simulink library "time_conversion_lib"  (R2016b)
settings: Solver=ode45  StartTime=0.0  StopTime=10.0  RelTol=1e-3  EnableMultiTasking=on
settings Model: Creator=Taylor  LastModifiedBy=taylorreynolds
settings DataIOCC: LimitDataPoints=on
settings OptimizationCC: LifeSpan=inf
settings DebuggingCC: AllowSymbolicDim=off  SFUnexpectedBacktrackingDiag=warning  SFNoUnconditionalDefaultTransitionDiag=warning  SFExecutionAtInitializationDiag=none
settings GRTTargetCC: TargetLangStandard=C89/C90 (ANSI)  GeneratePreprocessorConditionals=Disable all
settings ConfigComp: CovMetricSettings=dw  CovHtmlReporting=on  CovSaveCumulativeToWorkspaceVar=on  CovSaveSingleToWorkspaceVar=on  CovExternalEMLEnable=off

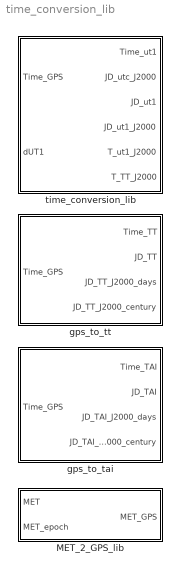
== system time_conversion_lib ==
  MET_2_GPS_lib : Subsystem
  gps_to_tai : Subsystem
  gps_to_tt : Subsystem
  time_conversion_lib : Subsystem

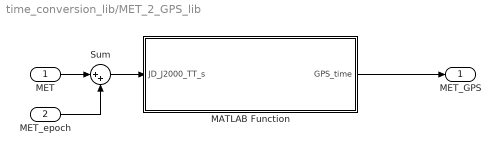
== system time_conversion_lib/MET_2_GPS_lib ==
  MET : Inport
  MET_epoch : Inport  Port=2
  MATLAB Function : MATLAB Function  TreatAsAtomicUnit=on
  Sum : Sum  Inputs=|++
  MET_GPS : Outport
  wires:
  MATLAB Function/1(GPS_time) -> MET_GPS/1
  MET/1 -> Sum/1
  MET_epoch/1 -> Sum/2
  Sum/1 -> MATLAB Function/1(JD_J2000_TT_s)

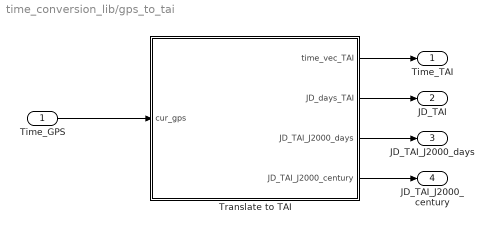
== system time_conversion_lib/gps_to_tai ==
  Time_GPS : Inport
  Translate to TAI : MATLAB Function  TreatAsAtomicUnit=on
  Time_TAI : Outport
  JD_TAI : Outport  Port=2
  JD_TAI_J2000_days : Outport  Port=3
  JD_TAI_J2000_century : Outport  Port=4
  wires:
  Translate to TAI/3(JD_TAI_J2000_days) -> JD_TAI_J2000_days/1
  Time_GPS/1 -> Translate to TAI/1(cur_gps)
  Translate to TAI/1(time_vec_TAI) -> Time_TAI/1
  Translate to TAI/2(JD_days_TAI) -> JD_TAI/1
  Translate to TAI/4(JD_TAI_J2000_century) -> JD_TAI_J2000_century/1

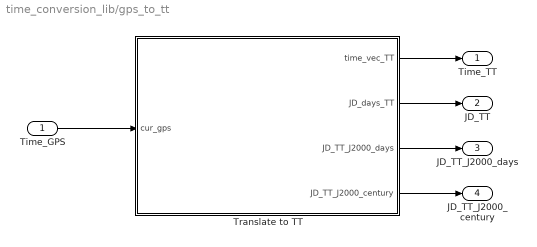
== system time_conversion_lib/gps_to_tt ==
  Time_GPS : Inport
  Translate to TT : MATLAB Function  TreatAsAtomicUnit=on
  Time_TT : Outport
  JD_TT : Outport  Port=2
  JD_TT_J2000_days : Outport  Port=3
  JD_TT_J2000_century : Outport  Port=4
  wires:
  Time_GPS/1 -> Translate to TT/1(cur_gps)
  Translate to TT/1(time_vec_TT) -> Time_TT/1
  Translate to TT/2(JD_days_TT) -> JD_TT/1
  Translate to TT/3(JD_TT_J2000_days) -> JD_TT_J2000_days/1
  Translate to TT/4(JD_TT_J2000_century) -> JD_TT_J2000_century/1

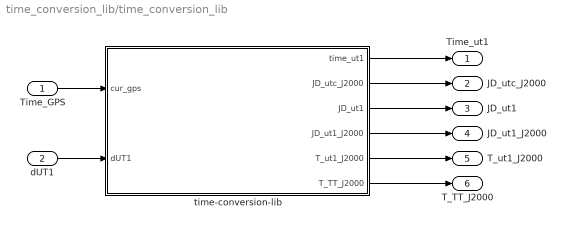
== system time_conversion_lib/time_conversion_lib ==
  Time_GPS : Inport
  dUT1 : Inport  Port=2
  time-conversion-lib : MATLAB Function  TreatAsAtomicUnit=on
  Time_ut1 : Outport
  JD_utc_J2000 : Outport  Port=2
  JD_ut1 : Outport  Port=3
  JD_ut1_J2000 : Outport  Port=4
  T_ut1_J2000 : Outport  Port=5
  T_TT_J2000 : Outport  Port=6
  wires:
  dUT1/1 -> time-conversion-lib/2(dUT1)
  time-conversion-lib/4(JD_ut1_J2000) -> JD_ut1_J2000/1
  Time_GPS/1 -> time-conversion-lib/1(cur_gps)
  time-conversion-lib/1(time_ut1) -> Time_ut1/1
  time-conversion-lib/5(T_ut1_J2000) -> T_ut1_J2000/1
  time-conversion-lib/3(JD_ut1) -> JD_ut1/1
  time-conversion-lib/6(T_TT_J2000) -> T_TT_J2000/1
  time-conversion-lib/2(JD_utc_J2000) -> JD_utc_J2000/1

== matlab function time_conversion_lib/gps_to_tai/Translate to TAI ==
  data: cur_gps input; time_vec_TAI output; JD_days_TAI output; JD_TAI_J2000_days output; JD_TAI_J2000_century output
function [time_vec_TAI,JD_days_TAI,JD_TAI_J2000_days,JD_TAI_J2000_century] = fcn(cur_gps)
% ----------------------------------------------------------------------- %
% Husky-Sat 1, ADCS Subsystem
% T. Reynolds -- 2.7.18
% 
% Convert a GPS time into date-time, Julian date and Julian century in the
% TAI frame. Accounts for leap seconds, and uses both the regular JD epoch
% and J2000.
%
% #codegen
% ------ Constants ------ %
% Account for dUT1 to get closest estimate to UT1
%   dUT1 obtained from:
%       http://maia.usno.navy.mil/ser7/finals.daily
% ----------------------------------------------------------------------- %

% Constants
gps2tai     = 19; % Account for leap seconds GPS --> TAI
sec2day     = 1/86400; 
day2sec     = 86400;
week2day    = 7;
JD_1900     = 2415019.5;
JD_GPSepoch = 2444244.5;
JD_J2000    = 2451545.0;
JD2cent     = 1/36525;
Lmonth      = [31, 28, 31, 30, 31, 30, 31, 31, 30, 31, 30, 31];

sec_in = cur_gps(1); week_in = cur_gps(2);
% --------------------------- %

% Translate GPS w-s to JD and Gregorian ymd-hms
JD_days_gps     = JD_GPSepoch + week2day*week_in + sec2day*sec_in;
JD_days_TAI     = JD_days_gps + sec2JD*gps2tai;

JD_TAI_J2000_days       = JD_days_TAI - JD_J2000;
JD_TAI_J2000_century    = JD_TAI_J2000_days*JD2cent;

T1900   = (JD_days_TAI - JD_1900)/365.25;

year    = 1900 + floor(T1900);

leapyrs     = floor((year - 1900 - 1)*0.25);
days    = (JD_days_TAI - JD_1900) - ((year - 1900)*365 + leapyrs );

if days < 1
    year = year - 1;
    leapyrs = floor((year - 1900 - 1)*0.25);
    days    = (JD_days_TAI - JD_1900) - ((year - 1900)*365 + leapyrs );
end

if mod(year,4) == 0
    Lmonth(2) = 29;
end

dayofyear   = floor(days);

day     = 0;
month   = 0;

while day < dayofyear
    month   = month + 1;
    day = day + Lmonth(month);
end

%dayofmonth = dayofyear - (day - Lmonth(month));

tau     = 24*( day - dayofyear );

hour    = floor( tau );
min     = floor( 60*(tau - hour) );
sec     = 3600*( tau - hour - (min/60) );

time_vec_TAI = [year,month,day,hour,min,sec];

== matlab function time_conversion_lib/time-conversion-lib ==
  data: time_ut1 output; JD_utc_J2000 output; cur_gps input; JD_ut1 output; JD_ut1_J2000 output; T_ut1_J2000 output; dUT1 input; T_TT_J2000 output
function [time_ut1,JD_utc_J2000,JD_ut1,JD_ut1_J2000,T_ut1_J2000,T_TT_J2000] = fcn(cur_gps,dUT1)
% ----------------------------------------------------------------------- %
% Husky-Sat 1, ADCS Subsystem
% 
% Convert a GPS time into date-time, Julian date and Julian century in the
% UT1 and TT frames. Accounts for leap seconds.
%
%   dUT1 obtained from:
%       http://maia.usno.navy.mil/ser7/finals.daily
%
% T. Reynolds -- 2.28.18
% ----------------------------------------------------------------------- %
% #codegen

% Constants
dAT         = 37.0;     % From MJD 58158 (Feb 7, 2018)
gps2tai     = 19.0;     % From MJD 58158
gps2tt      = 32.184 + gps2tai;
gps2utc     = gps2tai - dAT;
gps2ut1     = gps2tai - dAT + dUT1;
sec2day     = 1/86400; 
week2day    = 7;
JD_GPSepoch = 2444244.5;
JD_J2000    = 2451545.0;
JD2cent     = 1/36525;

sec_in = cur_gps(1); week_in = cur_gps(2);
% --------------------------- %

% Translate GPS w-s to JD and Gregorian ymd-hms
JD_days_gps     = JD_GPSepoch + week2day*week_in + sec2day*sec_in;
JD_utc          = JD_days_gps + sec2day*gps2utc;
JD_ut1          = JD_days_gps + sec2day*gps2ut1;
JD_TT           = JD_days_gps + sec2day*gps2tt;

JD_utc_J2000    = JD_utc - JD_J2000;
JD_ut1_J2000    = JD_ut1 - JD_J2000;
T_ut1_J2000     = JD_ut1_J2000*JD2cent;
T_TT_J2000      = JD2cent*( JD_TT - JD_J2000 );

time_ut1 = JD_2_ymdhms( JD_ut1 );

end

function [time] = JD_2_ymdhms( JD )
% This algorithm is based on Vallado 4e algorithm 22, pp 202.

% Constants
JD_1900     = 2415019.5;
Lmonth      = [31, 28, 31, 30, 31, 30, 31, 31, 30, 31, 30, 31];

% Convert JD to date-time
T1900   = (JD - JD_1900)/365.25; % base epoch is 1900
year    = 1900 + floor(T1900);

leapyrs = floor((year - 1900 - 1)*0.25);
days    = (JD - JD_1900) - ((year - 1900)*365 + leapyrs );

if days < 1
    year    = year - 1;
    leapyrs = floor((year - 1900 - 1)*0.25);
    days    = (JD - JD_1900) - ((year - 1900)*365 + leapyrs );
end

if mod(year,4) == 0
    Lmonth(2) = 29;
end

dayofyear   = floor(days);

day     = 0;
month   = 0;

while day < dayofyear
    month   = month + 1;
    day = day + Lmonth(month);
end

%dayofmonth = dayofyear - (day - Lmonth(month));

tau     = 24*( days-dayofyear );
hour    = floor( tau );
min     = floor( 60*(tau - hour) );
sec     = 3600*( tau - hour - (min/60) );

time    = [ year, month, dayofyear, hour, min, sec ];
end

== matlab function time_conversion_lib/MET_2_GPS_lib/MATLAB Function ==
  data: JD_J2000_TT_s input; GPS_time output
function GPS_time   = JDTT_2_GPS( JD_J2000_TT_s )
% ----------------------------------------------------------------------- %
% Husky-Sat 1, ADCS Subsystem
% 
% Convert a JD_J2000_TT in seconds into the GPS epoch and SoW-Week format.
%
%
% T. Reynolds -- 3.9.18
% ----------------------------------------------------------------------- %
% #codegen

% Constants
gps2tai     = 19.0;     % From MJD 58158
gps2tt      = 32.184 + gps2tai;
day2sec     = 86400; 
sec2day     = 1/day2sec;
dayinweek   = 7;
JD_GPSepoch = 2444244.5;
JD_J2000    = 2451545.0;

% Map input to JD_J2000_TT_days
JD_J2000_TT     = JD_J2000_TT_s * sec2day;

% Map input to GPS time frame
JD_J2000_GPS    = JD_J2000_TT - sec2day*gps2tt;
JD_GPS          = JD_J2000_GPS + JD_J2000;
JD_GPS_since_epoch    = JD_GPS - JD_GPSepoch;

% Convert to SoW and Week
week    = floor(JD_GPS_since_epoch/dayinweek);

sec_of_week    = day2sec * (JD_GPS_since_epoch - week*dayinweek);

GPS_time = [ sec_of_week; week ];

end

== matlab function time_conversion_lib/gps_to_tt/Translate to TT ==
  data: cur_gps input; time_vec_TT output; JD_days_TT output; JD_TT_J2000_days output; JD_TT_J2000_century output
function [time_vec_TT,JD_days_TT,JD_TT_J2000_days,JD_TT_J2000_century] = fcn(cur_gps)
% ----------------------------------------------------------------------- %
% Husky-Sat 1, ADCS Subsystem
% T. Reynolds -- 2.7.18
% 
% Convert a GPS time into date-time, Julian date and Julian century in the
% TT frame. Accounts for leap seconds, and uses both the regular JD epoch
% and J2000.
%
% #codegen
% ------ Constants ------ %
% Account for dUT1 to get closest estimate to UT1
%   dUT1 obtained from:
%       http://maia.usno.navy.mil/ser7/finals.daily
% ----------------------------------------------------------------------- %

% Constants
gps2tai     = 19.0;
gps2tt      = 32.184 + gps2tai;
sec2day     = 1/86400; 
day2sec     = 86400;
week2day    = 7;
JD_1900     = 2415019.5;
JD_GPSepoch = 2444244.5;
JD_J2000    = 2451545.0;
JD2cent     = 1/36525;
Lmonth      = [31, 28, 31, 30, 31, 30, 31, 31, 30, 31, 30, 31];

sec_in = cur_gps(1); week_in = cur_gps(2);

% Translate GPS w-s to JD and Gregorian ymd-hms
JD_days_gps     = JD_GPSepoch + week2day*week_in + sec2day*sec_in;
JD_days_TT      = JD_days_gps + sec2day*gps2tt;

JD_TT_J2000_days       = JD_days_TT - JD_J2000;
JD_TT_J2000_century    = JD_TT_J2000_days*JD2cent;

% Convert JD to date-time
T1900   = (JD_days_TT - JD_1900)/365.25;
year    = 1900 + floor(T1900);

leapyrs     = floor((year - 1900 - 1)*0.25);
days    = (JD_days_TT - JD_1900) - ((year - 1900)*365 + leapyrs );

if days < 1
    year = year - 1;
    leapyrs = floor((year - 1900 - 1)*0.25);
    days    = (JD_days_TT - JD_1900) - ((year - 1900)*365 + leapyrs );
end

if mod(year,4) == 0
    Lmonth(2) = 29;
end

dayofyear   = floor(days);

day     = 0;
month   = 0;

while day < dayofyear
    month = month + 1;
    day = day + Lmonth(month);   
end

%dayofmonth = dayofyear - (day-Lmonth(month));

tau     = 24*( day - dayofyear );

hour    = floor( tau );
min     = floor( 60*(tau - hour) );
sec     = 3600*( tau - hour - (min/60) );

time_vec_TT = [year,month,day,hour,min,sec];
